simulink library "nist_library"  (R2012b)
settings: Solver=VariableStepDiscrete  StartTime=0  StopTime=1000  RelTol=1e-3
undefined symbols (not defined in the file or in its folder): sfp, xlipgetpartsetting
libraries: xbsIndex_r4 x128, xps_library x10, nist_library x5, casper_library_misc x2, casper_library_delays x1
(part 2 of 3)

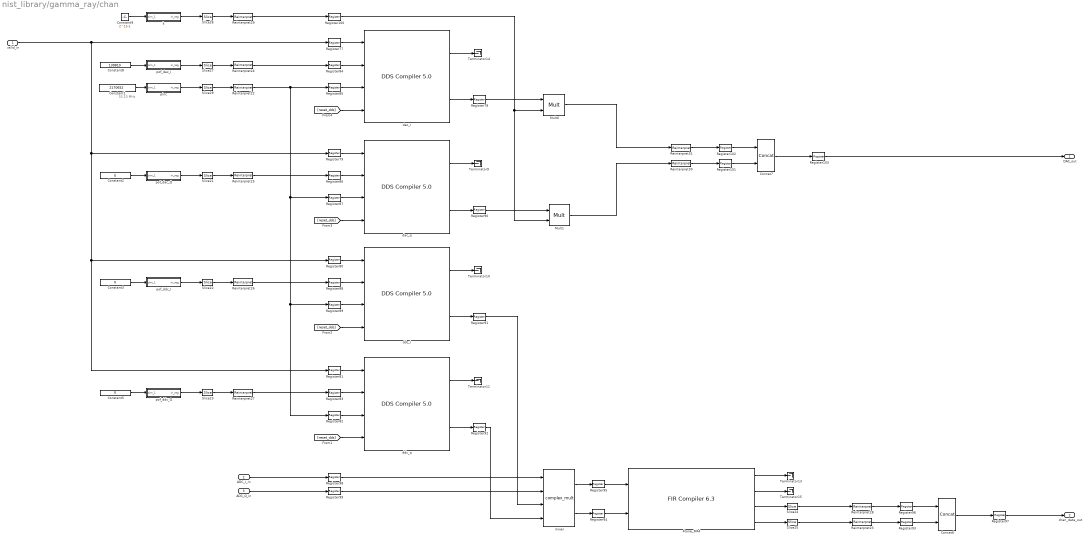
== system nist_library/gamma_ray/chan ==
  note: 33.10 MHz
  valid_in : Inport
  ADC_I_in : Inport  Port=2
  ADC_Q_in : Inport  Port=3
  4tone_FIR4 : xbsIndex_r4/FIR Compiler 6.3   coefficientvector=|  coefficient_sets=1  coefficient_reload=off  filter_type=Decimation  rate_change_type=Integer  interpolation_rate=1  decimation_rate=32  zero_pack_factor=1  channel_sequence=Basic  number_channels=1  pattern_list='P4-0,P4-1,P4-2,P4-3,P4-4'  number_paths=2  ratespecification=Maximum_Possible  sampleperiod=1  hardwareoversamplingrate=1  coefficient_sign=Signed  quantization=Maximize_Dynamic_Range  coefficient_width=14  bestprecision=on  coefficient_fractional_bits=19  coefficient_structure=Inferred  output_rounding_mode=Full_Precision  output_width=37  filter_architecture=Systolic_Multiply_Accumulate  optimization_goal=Speed  data_buffer_type=Automatic  coefficient_buffer_type=Automatic  input_buffer_type=Automatic  output_buffer_type=Automatic  preference_for_other_storage=Automatic  multi_column_support=Automatic  columnconfig='6'  inter_column_pipe_length=4  data_has_tlast=Not_Required  m_data_has_tready=off  s_data_has_fifo=off  s_data_has_tuser=Not_Required  m_data_has_tuser=Not_Required  s_config_sync_mode=On_Vector  s_config_method=Single  num_reload_slots=1  has_aclken=off  has_aresetn=off  infoeditControl=ARESETn must be asserted for a minimum of 2 cycles  trim_axipin_name=on  passband_min=0.0  passband_max=0.5  stopband_min=0.5  stopband_max=1.0  filter_selection=1  gui_behaviour=Sysgen_GUI  data_sign=Signed  data_width=16  data_fractional_bits=0  data_tuser_width=1  wrapper_available=true  ip_wrap_arbitrary_binary_point=true  ip_name=FIR Compiler  ip_version=6.3  dsptool_ready=true  ipcore_usecache=true  ipcore_useipmodelcache=true  ipcore_xco_need_fpga_part=true  port_translation_map={ 'aclken' => 'en', 'aresetn' => 'rst' }  run_core_at_system_period=true  ipcore_fpga_part=xlipgetpartsetting(gcb, {'virtex6', 'xc6vlx75t', '-3', 'ff784'})  block_type=fir_compiler_v6_3
      | [-0.004945576762396428,
      |   -0.0004342883057649687,
      |   -0.0004527757842562489,
      |   -0.00047135508794586133,
      |   -0.0004900760160352433,
      |   -0.0005088491202341634,
      |   -0.0005276998075326542,
      |   -0.000546547689892913,
      |   -0.0005654106976756595,
      |   -0.0005842536506410355,
      |   -0.0006030758678252529,
      |   -0.0006218519805181901,
      |   -0.0006405593109170567,
      |   -0.0006591567458735757,
      |   -0.0006776073739076259,
      |   -0.0006958986468812184,
      |   -0.0007140042099462066,
      |   -0.0007319006600209546,
      |   -0.0007495093972269049,
      |   -0.0007668271585960446,
      |   -0.0007837985973345622,
      |   -0.0008004847303040206,
      |   -0.000816558074371364,
      |   -0.0008326200345679305,
      |   -0.0008476890784144612,
      |   -0.0008625819845990018,
      |   -0.0008769170955610819,
      |   -0.0008905305577127275,
      |   -0.0009033656899299501,
      |   -0.0009156876002588938,
      |   -0.0009273520644178088,
      |   -0.0009382657988844351,
      |   -0.0009483110316064441,
      |   -0.0009574973347303523,
      |   -0.0009658333049719338,
      |   -0.0009733313313066214,
      |   -0.0009799587143928333,
      |   -0.0009856660600118781,
      |   -0.0009903926937808462,
      |   -0.0009940677596952641,
      |   -0.0009966598452596546,
      |   -0.000998153968519799,
      |   -0.000998593356035598,
      |   -0.0009979111825704338,
      |   -0.0009960294595758752,
      |   -0.0009926783563137058,
      |   -0.0009880436514076226,
      |   -0.000982031391898333,
      |   -0.0009746337113269129,
      |   -0.0009654980393360141,
      |   -0.0009551560082698979,
      |   -0.0009429957574212681,
      |   -0.0009294056596159474,
      |   -0.000914171602626857,
      |   -0.0008973503366857223,
      |   -0.000878942322437554,
      |   -0.000859007904965905,
      |   -0.0008375223708520817,
      |   -0.0008144740754976798,
      |   -0.0007898272475786514,
      |   -0.000763536797547961,
      |   -0.0007355014208217633,
      |   -0.0007055613466193147,
      |   -0.0006735396862409652,
      |   -0.0006392625855017414,
      |   -0.0006026653869321149,
      |   -0.0005638068586411848,
      |   -0.0005230595719924339,
      |   -0.0004809687403886442,
      |   -0.00043837704566643677,
      |   -0.00039560896213626615,
      |   -0.00035091342147599566,
      |   -0.00029119482633680816,
      |   -0.00024536833097263795,
      |   -0.0001906961065569639,
      |   -0.00013483102607781525,
      |   -0.00007690955909354745,
      |   -0.000016939572257551775,
      |   0.00004513495368569713,
      |   0.00010925887350151524,
      |   0.00017545824739311695,
      |   0.00024370647006966253,
      |   0.0003140097493414791,
      |   0.00038636169901666757,
      |   0.0004607657781277247,
      |   0.0005372061736658805,
      |   0.0006156568094935992,
      |   0.0006961175943544187,
      |   0.0007785853200736446,
      |   0.0008630788198892816,
      |   0.0009495445843636534,
      |   0.0010379964931242205,
      |   0.001128373604827996,
      |   0.0012207869406940261,
      |   0.0013147339335047488,
      |   0.0014113051117916689,
      |   0.0015088046287546986,
      |   0.0016086178618879032,
      |   0.001710374623684377,
      |   0.001813704207904973,
      |   0.001918476737258179,
      |   0.0020249986066717507,
      |   0.0021332426046828837,
      |   0.002243139281813915,
      |   0.0023545178342436524,
      |   0.002467311106773295,
      |   0.0025814917958775327,
      |   0.0026970805798065944,
      |   0.0028140764665559688,
      |   0.002932452736284891,
      |   0.003052149716212075,
      |   0.0031730589096328936,
      |   0.003295082974456467,
      |   0.0034181327776174643,
      |   0.0035422318687688874,
      |   0.0036673470602604937,
      |   0.003793474203475983,
      |   0.0039202919503391115,
      |   0.004047974298812806,
      |   0.004176310479278306,
      |   0.004305369824361406,
      |   0.004434823623226295,
      |   0.0045650237557334685,
      |   0.0046955130722802505,
      |   0.004826572927246175,
      |   0.00495798092373961,
      |   0.005089684001623189,
      |   0.005221568885099941,
      |   0.005353580377814376,
      |   0.005485579174458702,
      |   0.005617437626364228,
      |   0.005749047117597647,
      |   0.0058803760039980715,
      |   0.006011442594511834,
      |   0.006142272122013944,
      |   0.006272868641007802,
      |   0.0064031295153719504,
      |   0.006532863680215721,
      |   0.006661734821984142,
      |   0.006789525170342706,
      |   0.006916152986843038,
      |   0.0070421853694426426,
      |   0.007168266899850572,
      |   0.007294020325804492,
      |   0.0074148009918842,
      |   0.007538089119347543,
      |   0.007658471844329333,
      |   0.007777822658570999,
      |   0.007895704119665286,
      |   0.008012090275347652,
      |   0.008126861717259622,
      |   0.008239992610369232,
      |   0.008351384354342956,
      |   0.008460987880866197,
      |   0.008568730151338539,
      |   0.008674543678558294,
      |   0.008778340723400018,
      |   0.008880044308708633,
      |   0.008979602919157281,
      |   0.00907695323823665,
      |   0.00917204042884042,
      |   0.009264766789124777,
      |   0.009355105058699655,
      |   0.009442951431156595,
      |   0.009528293972594817,
      |   0.009610871314808363,
      |   0.009691496211636529,
      |   0.009767947553766466,
      |   0.009843401553078193,
      |   0.009915416541618427,
      |   0.009984126316499963,
      |   0.010050047903624215,
      |   0.010113422494991843,
      |   0.01017390543674861,
      |   0.010231296264840794,
      |   0.01028545119457461,
      |   0.010336421183108397,
      |   0.01038426038132455,
      |   0.010429014817948074,
      |   0.010470657332826963,
      |   0.01050912404868889,
      |   0.010544328818563124,
      |   0.01057618966061078,
      |   0.010604689751135063,
      |   0.010629849419136417,
      |   0.010651746091485394,
      |   0.010670350333632157,
      |   0.010685647353241094,
      |   0.010697494071983258,
      |   0.010706134504002181,
      |   0.010711226649567312,
      |   0.0107129982903304,
      |   0.010711226649567312,
      |   0.010706134504002181,
      |   0.010697494071983258,
      |   0.010685647353241094,
      |   0.010670350333632157,
      |   0.010651746091485394,
      |   0.010629849419136417,
      |   0.010604689751135063,
      |   0.01057618966061078,
      |   0.010544328818563124,
      |   0.01050912404868889,
      |   0.010470657332826963,
      |   0.010429014817948074,
      |   0.01038426038132455,
      |   0.010336421183108397,
      |   0.01028545119457461,
      |   0.010231296264840794,
      |   0.01017390543674861,
      |   0.010113422494991845,
      |   0.010050047903624215,
      |   0.009984126316499961,
      |   0.009915416541618425,
      |   0.009843401553078193,
      |   0.009767947553766466,
      |   0.009691496211636529,
      |   0.009610871314808363,
      |   0.009528293972594817,
      |   0.009442951431156595,
      |   0.009355105058699655,
      |   0.009264766789124777,
      |   0.00917204042884042,
      |   0.00907695323823665,
      |   0.008979602919157281,
      |   0.008880044308708633,
      |   0.008778340723400018,
      |   0.008674543678558294,
      |   0.008568730151338539,
      |   0.008460987880866197,
      |   0.008351384354342956,
      |   0.008239992610369232,
      |   0.008126861717259622,
      |   0.008012090275347652,
      |   0.007895704119665286,
      |   0.007777822658571,
      |   0.007658471844329333,
      |   0.007538089119347543,
      |   0.0074148009918842,
      |   0.007294020325804492,
      |   0.007168266899850572,
      |   0.0070421853694426426,
      |   0.006916152986843038,
      |   0.006789525170342706,
      |   0.006661734821984142,
      |   0.006532863680215721,
      |   0.0064031295153719504,
      |   0.006272868641007802,
      |   0.006142272122013944,
      |   0.006011442594511834,
      |   0.0058803760039980715,
      |   0.005749047117597647,
      |   0.005617437626364228,
      |   0.005485579174458702,
      |   0.005353580377814376,
      |   0.005221568885099941,
      |   0.005089684001623189,
      |   0.00495798092373961,
      |   0.004826572927246175,
      |   0.0046955130722802505,
      |   0.0045650237557334685,
      |   0.004434823623226295,
      |   0.004305369824361406,
      |   0.004176310479278306,
      |   0.004047974298812806,
      |   0.0039202919503391115,
      |   0.003793474203475983,
      |   0.0036673470602604937,
      |   0.0035422318687688874,
      |   0.0034181327776174647,
      |   0.003295082974456466,
      |   0.0031730589096328936,
      |   0.003052149716212075,
      |   0.002932452736284891,
      |   0.0028140764665559688,
      |   0.0026970805798065944,
      |   0.0025814917958775327,
      |   0.002467311106773295,
      |   0.0023545178342436524,
      |   0.002243139281813915,
      |   0.0021332426046828837,
      |   0.0020249986066717507,
      |   0.0019184767372581789,
      |   0.0018137042079049725,
      |   0.001710374623684377,
      |   0.0016086178618879032,
      |   0.0015088046287546986,
      |   0.0014113051117916689,
      |   0.0013147339335047488,
      |   0.0012207869406940261,
      |   0.001128373604827996,
      |   0.0010379964931242205,
      |   0.0009495445843636534,
      |   0.0008630788198892816,
      |   0.0007785853200736446,
      |   0.0006961175943544187,
      |   0.0006156568094935992,
      |   0.0005372061736658805,
      |   0.0004607657781277247,
      |   0.00038636169901666757,
      |   0.0003140097493414791,
      |   0.00024370647006966253,
      |   0.000175458247393117,
      |   0.00010925887350151526,
      |   0.000045134953685697144,
      |   -0.000016939572257551775,
      |   -0.00007690955909354741,
      |   -0.00013483102607781503,
      |   -0.0001906961065569639,
      |   -0.00024536833097263795,
      |   -0.00029119482633680816,
      |   -0.0003509134214759956,
      |   -0.00039560896213626615,
      |   -0.00043837704566643677,
      |   -0.0004809687403886442,
      |   -0.0005230595719924339,
      |   -0.0005638068586411848,
      |   -0.0006026653869321149,
      |   -0.0006392625855017414,
      |   -0.0006735396862409652,
      |   -0.0007055613466193147,
      |   -0.0007355014208217633,
      |   -0.000763536797547961,
      |   -0.000789827247578651,
      |   -0.0008144740754976798,
      |   -0.0008375223708520817,
      |   -0.000859007904965905,
      |   -0.000878942322437554,
      |   -0.0008973503366857223,
      |   -0.000914171602626857,
      |   -0.0009294056596159474,
      |   -0.0009429957574212681,
      |   -0.0009551560082698979,
      |   -0.0009654980393360141,
      |   -0.0009746337113269129,
      |   -0.000982031391898333,
      |   -0.0009880436514076226,
      |   -0.0009926783563137065,
      |   -0.0009960294595758755,
      |   -0.0009979111825704338,
      |   -0.000998593356035598,
      |   -0.0009981539685197994,
      |   -0.0009966598452596546,
      |   -0.0009940677596952641,
      |   -0.0009903926937808462,
      |   -0.000985666060011878,
      |   -0.0009799587143928333,
      |   -0.0009733313313066214,
      |   -0.0009658333049719338,
      |   -0.0009574973347303529,
      |   -0.0009483110316064446,
      |   -0.0009382657988844346,
      |   -0.0009273520644178088,
      |   -0.0009156876002588938,
      |   -0.0009033656899299501,
      |   -0.0008905305577127275,
      |   -0.0008769170955610819,
      |   -0.0008625819845990029,
      |   -0.0008476890784144612,
      |   -0.0008326200345679302,
      |   -0.000816558074371364,
      |   -0.0008004847303040206,
      |   -0.0007837985973345619,
      |   -0.0007668271585960446,
      |   -0.0007495093972269048,
      |   -0.0007319006600209546,
      |   -0.000714004209946207,
      |   -0.0006958986468812184,
      |   -0.0006776073739076259,
      |   -0.0006591567458735757,
      |   -0.0006405593109170567,
      |   -0.0006218519805181902,
      |   -0.0006030758678252529,
      |   -0.0005842536506410353,
      |   -0.0005654106976756595,
      |   -0.000546547689892913,
      |   -0.0005276998075326542,
      |   -0.0005088491202341634,
      |   -0.0004900760160352433,
      |   -0.00047135508794586133,
      |   -0.0004527757842562489,
      |   -0.0004342883057649687,
      |   -0.004945576762396428]
      settings: infoedit=Maximum Possible : Maximizes oversampling rate. Abstracted input handshake (no s_data_tvalid) and automatic rate propagation.<br>Hardware Oversampling Rate : Specifies oversampling rate relative to the input sample period. Abstracted input handshake (no s_data_tvalid) and automatic rate propagation.<br>Sample Period : Specifies absolute oversampling rate. No input handshake abstraction (exposes s_data_tvalid) and no rate propagation.
  Concat6 : xbsIndex_r4/Concat  num_inputs=2  dbl_ovrd=off  block_type=concat
  Concat7 : xbsIndex_r4/Concat  num_inputs=2  dbl_ovrd=off  block_type=concat
  Constant1 : Constant  Value=2170652
  Constant2 : Constant  Value=0
  Constant3 : Constant  Value=0
  Constant5 : Constant  Value=0
  Constant8 : Constant  Value=139810
  Constant9 : Constant  Value=2^15-1
  Mult0 : xbsIndex_r4/Mult  precision=User Defined  arith_type="Signed  (2's comp)"  n_bits=16  bin_pt=15  quantization=Truncate  overflow=Wrap  en=off  latency=4  dbl_ovrd=off  use_behavioral_HDL=off  opt=Speed  use_embedded=on  optimum_pipeline=off  pipeline=on  use_rpm=on  placement_style=Triangular  block_type=mult
  Mult1 : xbsIndex_r4/Mult  precision=User Defined  arith_type="Signed  (2's comp)"  n_bits=16  bin_pt=15  quantization=Truncate  overflow=Wrap  en=off  latency=4  dbl_ovrd=off  use_behavioral_HDL=off  opt=Speed  use_embedded=on  optimum_pipeline=off  pipeline=on  use_rpm=on  placement_style=Triangular  block_type=mult
  Register{77..103} (27 alike) : xbsIndex_r4/Register  init=0  rst=off  en=off  dbl_ovrd=off  block_type=register
  Reinterpret{22,24..27} (5 alike) : xbsIndex_r4/Reinterpret  force_arith_type=on  arith_type="Signed  (2's comp)"  force_bin_pt=on  bin_pt=24  block_type=reinterpret
      settings: block_version=10.1.3
  Reinterpret{23,28,30..31} (4 alike) : xbsIndex_r4/Reinterpret  force_arith_type=on  arith_type=Unsigned  force_bin_pt=on  bin_pt=0  block_type=reinterpret
      settings: block_version=10.1.3
  Reinterpret29 : xbsIndex_r4/Reinterpret  force_arith_type=on  arith_type="Signed  (2's comp)"  force_bin_pt=on  bin_pt=15  block_type=reinterpret
      settings: block_version=10.1.3
  Slice{21..23,27,29} (5 alike) : xbsIndex_r4/Slice  nbits=24  boolean_output=off  mode=Lower Bit Location + Width  bit1=0  base1=MSB of Input  bit0=0  base0=LSB of Input  dbl_ovrd=off  block_type=slice
      settings: block_version=10.1.3
  Slice24 : xbsIndex_r4/Slice  nbits=32  boolean_output=off  mode=Two Bit Locations  bit1=2  base1=Binary Point of Input  bit0=-16  base0=Binary Point of Input  dbl_ovrd=off  block_type=slice
      settings: block_version=10.1.3
  Slice25 : xbsIndex_r4/Slice  nbits=32  boolean_output=off  mode=Two Bit Locations  bit1=2  base1=Binary Point of Input  bit0=-16  base0=Binary Point of Input  dbl_ovrd=off  block_type=slice
      settings: block_version=10.1.3
  Slice26 : xbsIndex_r4/Slice  nbits=16  boolean_output=off  mode=Lower Bit Location + Width  bit1=0  base1=MSB of Input  bit0=0  base0=LSB of Input  dbl_ovrd=off  block_type=slice
      settings: block_version=10.1.3
  Terminator{9..11,13..15} (6 alike) : Terminator
  dac_I : xbsIndex_r4/DDS Compiler 5.0   partspresent=Phase_Generator_and_SIN_COS_LUT  dds_clock_rate=256  channels=1  parameter_entry=Hardware_Parameters  spurious_free_dynamic_range=36  frequency_resolution=0.4  noise_shaping=None  phase_width=24  output_width=16  output_selection=Cosine  negative_sine=off  negative_cosine=off  amplitude_mode=Full_Range  memory_type=Auto  optimization_goal=Speed  dsp48_use=Maximal  latency_configuration=Auto  latency=5  has_phase_out=off  has_aclken=off  has_aresetn=on  explicit_period=off  period=1  data_has_tlast=Not_Required  has_tready=off  s_phase_has_tuser=Not_Required  m_data_has_tuser=Not_Required  m_phase_has_tuser=Not_Required  s_phase_tuser_width=1  s_config_sync_mode=On_Vector  phase_increment=Programmable  output_frequency1=0  output_frequency2=0  output_frequency3=0  output_frequency4=0  output_frequency5=0  output_frequency6=0  output_frequency7=0  output_frequency8=0  output_frequency9=0  output_frequency10=0  output_frequency11=0  output_frequency12=0  output_frequency13=0  output_frequency14=0  output_frequency15=0  output_frequency16=0  pinc1='1101000110110'  pinc2='0'  pinc3='0'  pinc4='0'  pinc5='0'  pinc6='0'  pinc7='0'  pinc8='0'  pinc9='0'  pinc10='0'  pinc11='0'  pinc12='0'  pinc13='0'  pinc14='0'  pinc15='0'  pinc16='0'  phase_offset=Programmable  phase_offset_angles1=0  phase_offset_angles2=0  phase_offset_angles3=0  phase_offset_angles4=0  phase_offset_angles5=0  phase_offset_angles6=0  phase_offset_angles7=0  phase_offset_angles8=0  phase_offset_angles9=0  phase_offset_angles10=0  phase_offset_angles11=0  phase_offset_angles12=0  phase_offset_angles13=0  phase_offset_angles14=0  phase_offset_angles15=0  phase_offset_angles16=0  poff1='0'  poff2='0'  poff3='0'  poff4='0'  poff5='0'  poff6='0'  poff7='0'  poff8='0'  poff9='0'  poff10='0'  poff11='0'  poff12='0'  poff13='0'  poff14='0'  poff15='0'  poff16='0'  trim_axipin_name=on  por_mode=false  gui_behaviour=Sysgen  ip_name=DDS Compiler  ip_version=5.0  dsptool_ready=true  wrapper_available=true  port_translation_map={ 'aclken' => 'en', 'aresetn' => 'rst' }  ipcore_xco_need_fpga_part=true  ipcore_fpga_part=xlipgetpartsetting(gcb, {'virtex6', 'xc6vlx75t', '-3', 'ff784'})  ipcore_usecache=true  ipcore_useipmodelcache=true  ipcore_verbose=false  block_type=dds_compiler_v5_0
  dac_q : xbsIndex_r4/DDS Compiler 5.0   partspresent=Phase_Generator_and_SIN_COS_LUT  dds_clock_rate=256  channels=1  parameter_entry=Hardware_Parameters  spurious_free_dynamic_range=36  frequency_resolution=0.4  noise_shaping=None  phase_width=24  output_width=16  output_selection=Cosine  negative_sine=off  negative_cosine=off  amplitude_mode=Full_Range  memory_type=Auto  optimization_goal=Speed  dsp48_use=Maximal  latency_configuration=Auto  latency=5  has_phase_out=off  has_aclken=off  has_aresetn=on  explicit_period=off  period=1  data_has_tlast=Not_Required  has_tready=off  s_phase_has_tuser=Not_Required  m_data_has_tuser=Not_Required  m_phase_has_tuser=Not_Required  s_phase_tuser_width=1  s_config_sync_mode=On_Vector  phase_increment=Programmable  output_frequency1=0  output_frequency2=0  output_frequency3=0  output_frequency4=0  output_frequency5=0  output_frequency6=0  output_frequency7=0  output_frequency8=0  output_frequency9=0  output_frequency10=0  output_frequency11=0  output_frequency12=0  output_frequency13=0  output_frequency14=0  output_frequency15=0  output_frequency16=0  pinc1='1101000110110'  pinc2='0'  pinc3='0'  pinc4='0'  pinc5='0'  pinc6='0'  pinc7='0'  pinc8='0'  pinc9='0'  pinc10='0'  pinc11='0'  pinc12='0'  pinc13='0'  pinc14='0'  pinc15='0'  pinc16='0'  phase_offset=Programmable  phase_offset_angles1=0  phase_offset_angles2=0  phase_offset_angles3=0  phase_offset_angles4=0  phase_offset_angles5=0  phase_offset_angles6=0  phase_offset_angles7=0  phase_offset_angles8=0  phase_offset_angles9=0  phase_offset_angles10=0  phase_offset_angles11=0  phase_offset_angles12=0  phase_offset_angles13=0  phase_offset_angles14=0  phase_offset_angles15=0  phase_offset_angles16=0  poff1='0'  poff2='0'  poff3='0'  poff4='0'  poff5='0'  poff6='0'  poff7='0'  poff8='0'  poff9='0'  poff10='0'  poff11='0'  poff12='0'  poff13='0'  poff14='0'  poff15='0'  poff16='0'  trim_axipin_name=on  por_mode=false  gui_behaviour=Sysgen  ip_name=DDS Compiler  ip_version=5.0  dsptool_ready=true  wrapper_available=true  port_translation_map={ 'aclken' => 'en', 'aresetn' => 'rst' }  ipcore_xco_need_fpga_part=true  ipcore_fpga_part=xlipgetpartsetting(gcb, {'virtex6', 'xc6vlx75t', '-3', 'ff784'})  ipcore_usecache=true  ipcore_useipmodelcache=true  ipcore_verbose=false  block_type=dds_compiler_v5_0
  ddc_I : xbsIndex_r4/DDS Compiler 5.0   partspresent=Phase_Generator_and_SIN_COS_LUT  dds_clock_rate=256  channels=1  parameter_entry=Hardware_Parameters  spurious_free_dynamic_range=36  frequency_resolution=0.4  noise_shaping=None  phase_width=24  output_width=12  output_selection=Cosine  negative_sine=off  negative_cosine=off  amplitude_mode=Full_Range  memory_type=Auto  optimization_goal=Speed  dsp48_use=Maximal  latency_configuration=Auto  latency=9  has_phase_out=off  has_aclken=off  has_aresetn=on  explicit_period=off  period=1  data_has_tlast=Not_Required  has_tready=off  s_phase_has_tuser=Not_Required  m_data_has_tuser=Not_Required  m_phase_has_tuser=Not_Required  s_phase_tuser_width=1  s_config_sync_mode=On_Vector  phase_increment=Programmable  output_frequency1=0  output_frequency2=0  output_frequency3=0  output_frequency4=0  output_frequency5=0  output_frequency6=0  output_frequency7=0  output_frequency8=0  output_frequency9=0  output_frequency10=0  output_frequency11=0  output_frequency12=0  output_frequency13=0  output_frequency14=0  output_frequency15=0  output_frequency16=0  pinc1='1101000110110'  pinc2='0'  pinc3='0'  pinc4='0'  pinc5='0'  pinc6='0'  pinc7='0'  pinc8='0'  pinc9='0'  pinc10='0'  pinc11='0'  pinc12='0'  pinc13='0'  pinc14='0'  pinc15='0'  pinc16='0'  phase_offset=Programmable  phase_offset_angles1=0  phase_offset_angles2=0  phase_offset_angles3=0  phase_offset_angles4=0  phase_offset_angles5=0  phase_offset_angles6=0  phase_offset_angles7=0  phase_offset_angles8=0  phase_offset_angles9=0  phase_offset_angles10=0  phase_offset_angles11=0  phase_offset_angles12=0  phase_offset_angles13=0  phase_offset_angles14=0  phase_offset_angles15=0  phase_offset_angles16=0  poff1='0'  poff2='0'  poff3='0'  poff4='0'  poff5='0'  poff6='0'  poff7='0'  poff8='0'  poff9='0'  poff10='0'  poff11='0'  poff12='0'  poff13='0'  poff14='0'  poff15='0'  poff16='0'  trim_axipin_name=on  por_mode=false  gui_behaviour=Sysgen  ip_name=DDS Compiler  ip_version=5.0  dsptool_ready=true  wrapper_available=true  port_translation_map={ 'aclken' => 'en', 'aresetn' => 'rst' }  ipcore_xco_need_fpga_part=true  ipcore_fpga_part=xlipgetpartsetting(gcb, {'virtex6', 'xc6vlx75t', '-3', 'ff784'})  ipcore_usecache=true  ipcore_useipmodelcache=true  ipcore_verbose=false  block_type=dds_compiler_v5_0
  ddc_q : xbsIndex_r4/DDS Compiler 5.0   partspresent=Phase_Generator_and_SIN_COS_LUT  dds_clock_rate=256  channels=1  parameter_entry=Hardware_Parameters  spurious_free_dynamic_range=36  frequency_resolution=0.4  noise_shaping=None  phase_width=24  output_width=12  output_selection=Cosine  negative_sine=off  negative_cosine=off  amplitude_mode=Full_Range  memory_type=Auto  optimization_goal=Speed  dsp48_use=Maximal  latency_configuration=Auto  latency=9  has_phase_out=off  has_aclken=off  has_aresetn=on  explicit_period=off  period=1  data_has_tlast=Not_Required  has_tready=off  s_phase_has_tuser=Not_Required  m_data_has_tuser=Not_Required  m_phase_has_tuser=Not_Required  s_phase_tuser_width=1  s_config_sync_mode=On_Vector  phase_increment=Programmable  output_frequency1=0  output_frequency2=0  output_frequency3=0  output_frequency4=0  output_frequency5=0  output_frequency6=0  output_frequency7=0  output_frequency8=0  output_frequency9=0  output_frequency10=0  output_frequency11=0  output_frequency12=0  output_frequency13=0  output_frequency14=0  output_frequency15=0  output_frequency16=0  pinc1='1101000110110'  pinc2='0'  pinc3='0'  pinc4='0'  pinc5='0'  pinc6='0'  pinc7='0'  pinc8='0'  pinc9='0'  pinc10='0'  pinc11='0'  pinc12='0'  pinc13='0'  pinc14='0'  pinc15='0'  pinc16='0'  phase_offset=Programmable  phase_offset_angles1=0  phase_offset_angles2=0  phase_offset_angles3=0  phase_offset_angles4=0  phase_offset_angles5=0  phase_offset_angles6=0  phase_offset_angles7=0  phase_offset_angles8=0  phase_offset_angles9=0  phase_offset_angles10=0  phase_offset_angles11=0  phase_offset_angles12=0  phase_offset_angles13=0  phase_offset_angles14=0  phase_offset_angles15=0  phase_offset_angles16=0  poff1='0'  poff2='0'  poff3='0'  poff4='0'  poff5='0'  poff6='0'  poff7='0'  poff8='0'  poff9='0'  poff10='0'  poff11='0'  poff12='0'  poff13='0'  poff14='0'  poff15='0'  poff16='0'  trim_axipin_name=on  por_mode=false  gui_behaviour=Sysgen  ip_name=DDS Compiler  ip_version=5.0  dsptool_ready=true  wrapper_available=true  port_translation_map={ 'aclken' => 'en', 'aresetn' => 'rst' }  ipcore_xco_need_fpga_part=true  ipcore_fpga_part=xlipgetpartsetting(gcb, {'virtex6', 'xc6vlx75t', '-3', 'ff784'})  ipcore_usecache=true  ipcore_useipmodelcache=true  ipcore_verbose=false  block_type=dds_compiler_v5_0
  k : Subsystem  Tag=xps:sw_reg  AncestorBlock=xps_library/software register  mask(swreg){mode=one value, io_dir=From Processor, io_delay=0, sample_period=1, names=reg, bitwidths=32, arith_types=0, bin_pts=0, sim_port=on, show_format=off}
      mask prompts: io_dir "I/O direction"; io_delay "I/O delay"; sample_period "Sample period"; names "Name:"; bitwidths "Bitwidth:"; arith_types "Type (ufix=0, fix=1, bool=2):"; bin_pts "Binary pt:"; sim_port "Provide sim input/output?"; show_format "Print format string?"
      mask init:
      | swreg_init(gcb)
      settings: AttributesFormatString=1input
      mask TypeOptions mode: one value | fields of equal size | fields of arbitrary size
      mask Callback mode: swreg_cb(gcb);
      mask TypeOptions io_dir: To Processor | From Processor
      mask Callback io_dir:
      | mask_enables = get_param(gcb, 'MaskEnables');
      | mask_names = get_param(gcb, 'MaskNames');
      | if strcmp(get_param(gcb, 'io_dir'), 'To Processor'),
      |     mask_enables{ismember(mask_names, 'sample_period')} = 'off';
      | else
      |     mask_enables{ismember(mask_names, 'sample_period')} = 'on';
      | end
      | set_param(gcb, 'MaskEnables', mask_enables);
      mask Callback bitwidths:
      | swreg_maskcheck(gcb);
      | % blk = gcb;
      | % mode = get_param(blk, 'mode');
      | % current_widths = eval(get_param(blk, 'bitwidths'));
      | % if (strcmp(mode, 'one value') || strcmp(mode, 'fields of equal size')) && (length(current_widths) > 1),
      | %     error('Only one width may be specified for this mode.');
      | % elseif strcmp(mode, 'fields of arbitrary size')
      | %     current_names = textscan(strtrim(strrep(strrep(get_param(blk, 'names'), ']', ''), '[', '')), '%s');
      | %     current_names = current_names{1};
      | %     numios = length(current_names);
      | %     if length(current_widths) ~= numios,
      | %         error('%d field names specified, but %d widths?', numios, length(current_widths));
      | %     end
      | % end
      | % total_width = 0;
      | % for ctr = 1 : length(current_widths),
      | %     total_width = total_width + current_widths(ctr);
      | % end
      | % if total_width > 32,
      | %     error('Total width must be 32 or less, set to %d.', total_width);
      | % end
      mask Callback arith_types:
      | [numios, ~, ~, ~, current_types] = swreg_maskcheck(gcb);
      | % blk = gcb;
      | % mode = get_param(blk, 'mode');
      | % current_types = eval(get_param(blk, 'arith_types'));
      | % numios = length(current_types);
      | % if (strcmp(mode, 'one value') || strcmp(mode, 'fields of equal size')) && (length(current_types) > 1),
      | %     error('Only one type may be specified for this mode.');
      | % elseif strcmp(mode, 'fields of arbitrary size')
      | %     current_names = textscan(strtrim(strrep(strrep(get_param(blk, 'names'), ']', ''), '[', '')), '%s');
      | %     current_names = current_names{1};
      | %     numios = length(current_names);
      | %     if length(current_types) ~= numios,
      | %         error('%d field names specified, but %d types?', numios, length(current_types));
      | %     end
      | % end
      | problem = 0;
      | for ctr = 1 : numios,
      |     t = current_types(ctr);
      |     if (t < 0) || (t > 2),
      |         problem = t;
      |         ctr = numios + 1;
      |     end
      | end
      | if problem ~= 0,
      |     error('Type cannot be %i, must be 0, 1 or 2.', problem);
      | end
      mask Callback bin_pts:
      | swreg_maskcheck(gcb);
      | % blk = gcb;
      | % mode = get_param(blk, 'mode');
      | % current_bins = eval(get_param(blk, 'bin_pts'));
      | % if (strcmp(mode, 'one value') || strcmp(mode, 'fields of equal size')) && (length(current_bins) > 1),
      | %     error('Only one binary pt may be specified for this mode.');
      | % elseif strcmp(mode, 'fields of arbitrary size')
      | %     current_names = textscan(strtrim(strrep(strrep(get_param(blk, 'names'), ']', ''), '[', '')), '%s');
      | %     current_names = current_names{1};
      | %     numios = length(current_names);
      | %     if length(current_bins) ~= numios,
      | %         error('%d field names specified, but %d binary pts?', numios, length(current_bins));
      | %     end
      | % end
  mixer : nist_library/complex_mult
  pinc : Subsystem  Tag=xps:sw_reg  AncestorBlock=xps_library/software register  mask(swreg){mode=one value, io_dir=From Processor, io_delay=0, sample_period=1, names=reg, bitwidths=32, arith_types=0, bin_pts=0, sim_port=on, show_format=off}
      mask prompts: io_dir "I/O direction"; io_delay "I/O delay"; sample_period "Sample period"; names "Name:"; bitwidths "Bitwidth:"; arith_types "Type (ufix=0, fix=1, bool=2):"; bin_pts "Binary pt:"; sim_port "Provide sim input/output?"; show_format "Print format string?"
      mask init:
      | swreg_init(gcb)
      settings: AttributesFormatString=1input
      mask TypeOptions mode: one value | fields of equal size | fields of arbitrary size
      mask Callback mode: swreg_cb(gcb);
      mask TypeOptions io_dir: To Processor | From Processor
      mask Callback io_dir:
      | mask_enables = get_param(gcb, 'MaskEnables');
      | mask_names = get_param(gcb, 'MaskNames');
      | if strcmp(get_param(gcb, 'io_dir'), 'To Processor'),
      |     mask_enables{ismember(mask_names, 'sample_period')} = 'off';
      | else
      |     mask_enables{ismember(mask_names, 'sample_period')} = 'on';
      | end
      | set_param(gcb, 'MaskEnables', mask_enables);
      mask Callback bitwidths:
      | swreg_maskcheck(gcb);
      | % blk = gcb;
      | % mode = get_param(blk, 'mode');
      | % current_widths = eval(get_param(blk, 'bitwidths'));
      | % if (strcmp(mode, 'one value') || strcmp(mode, 'fields of equal size')) && (length(current_widths) > 1),
      | %     error('Only one width may be specified for this mode.');
      | % elseif strcmp(mode, 'fields of arbitrary size')
      | %     current_names = textscan(strtrim(strrep(strrep(get_param(blk, 'names'), ']', ''), '[', '')), '%s');
      | %     current_names = current_names{1};
      | %     numios = length(current_names);
      | %     if length(current_widths) ~= numios,
      | %         error('%d field names specified, but %d widths?', numios, length(current_widths));
      | %     end
      | % end
      | % total_width = 0;
      | % for ctr = 1 : length(current_widths),
      | %     total_width = total_width + current_widths(ctr);
      | % end
      | % if total_width > 32,
      | %     error('Total width must be 32 or less, set to %d.', total_width);
      | % end
      mask Callback arith_types:
      | [numios, ~, ~, ~, current_types] = swreg_maskcheck(gcb);
      | % blk = gcb;
      | % mode = get_param(blk, 'mode');
      | % current_types = eval(get_param(blk, 'arith_types'));
      | % numios = length(current_types);
      | % if (strcmp(mode, 'one value') || strcmp(mode, 'fields of equal size')) && (length(current_types) > 1),
      | %     error('Only one type may be specified for this mode.');
      | % elseif strcmp(mode, 'fields of arbitrary size')
      | %     current_names = textscan(strtrim(strrep(strrep(get_param(blk, 'names'), ']', ''), '[', '')), '%s');
      | %     current_names = current_names{1};
      | %     numios = length(current_names);
      | %     if length(current_types) ~= numios,
      | %         error('%d field names specified, but %d types?', numios, length(current_types));
      | %     end
      | % end
      | problem = 0;
      | for ctr = 1 : numios,
      |     t = current_types(ctr);
      |     if (t < 0) || (t > 2),
      |         problem = t;
      |         ctr = numios + 1;
      |     end
      | end
      | if problem ~= 0,
      |     error('Type cannot be %i, must be 0, 1 or 2.', problem);
      | end
      mask Callback bin_pts:
      | swreg_maskcheck(gcb);
      | % blk = gcb;
      | % mode = get_param(blk, 'mode');
      | % current_bins = eval(get_param(blk, 'bin_pts'));
      | % if (strcmp(mode, 'one value') || strcmp(mode, 'fields of equal size')) && (length(current_bins) > 1),
      | %     error('Only one binary pt may be specified for this mode.');
      | % elseif strcmp(mode, 'fields of arbitrary size')
      | %     current_names = textscan(strtrim(strrep(strrep(get_param(blk, 'names'), ']', ''), '[', '')), '%s');
      | %     current_names = current_names{1};
      | %     numios = length(current_names);
      | %     if length(current_bins) ~= numios,
      | %         error('%d field names specified, but %d binary pts?', numios, length(current_bins));
      | %     end
      | % end
  pof_dac_I : Subsystem  Tag=xps:sw_reg  AncestorBlock=xps_library/software register  mask(swreg){mode=one value, io_dir=From Processor, io_delay=0, sample_period=1, names=reg, bitwidths=32, arith_types=0, bin_pts=0, sim_port=on, show_format=off}
      mask prompts: io_dir "I/O direction"; io_delay "I/O delay"; sample_period "Sample period"; names "Name:"; bitwidths "Bitwidth:"; arith_types "Type (ufix=0, fix=1, bool=2):"; bin_pts "Binary pt:"; sim_port "Provide sim input/output?"; show_format "Print format string?"
      mask init:
      | swreg_init(gcb)
      settings: AttributesFormatString=1input
      mask TypeOptions mode: one value | fields of equal size | fields of arbitrary size
      mask Callback mode: swreg_cb(gcb);
      mask TypeOptions io_dir: To Processor | From Processor
      mask Callback io_dir:
      | mask_enables = get_param(gcb, 'MaskEnables');
      | mask_names = get_param(gcb, 'MaskNames');
      | if strcmp(get_param(gcb, 'io_dir'), 'To Processor'),
      |     mask_enables{ismember(mask_names, 'sample_period')} = 'off';
      | else
      |     mask_enables{ismember(mask_names, 'sample_period')} = 'on';
      | end
      | set_param(gcb, 'MaskEnables', mask_enables);
      mask Callback bitwidths:
      | swreg_maskcheck(gcb);
      | % blk = gcb;
      | % mode = get_param(blk, 'mode');
      | % current_widths = eval(get_param(blk, 'bitwidths'));
      | % if (strcmp(mode, 'one value') || strcmp(mode, 'fields of equal size')) && (length(current_widths) > 1),
      | %     error('Only one width may be specified for this mode.');
      | % elseif strcmp(mode, 'fields of arbitrary size')
      | %     current_names = textscan(strtrim(strrep(strrep(get_param(blk, 'names'), ']', ''), '[', '')), '%s');
      | %     current_names = current_names{1};
      | %     numios = length(current_names);
      | %     if length(current_widths) ~= numios,
      | %         error('%d field names specified, but %d widths?', numios, length(current_widths));
      | %     end
      | % end
      | % total_width = 0;
      | % for ctr = 1 : length(current_widths),
      | %     total_width = total_width + current_widths(ctr);
      | % end
      | % if total_width > 32,
      | %     error('Total width must be 32 or less, set to %d.', total_width);
      | % end
      mask Callback arith_types:
      | [numios, ~, ~, ~, current_types] = swreg_maskcheck(gcb);
      | % blk = gcb;
      | % mode = get_param(blk, 'mode');
      | % current_types = eval(get_param(blk, 'arith_types'));
      | % numios = length(current_types);
      | % if (strcmp(mode, 'one value') || strcmp(mode, 'fields of equal size')) && (length(current_types) > 1),
      | %     error('Only one type may be specified for this mode.');
      | % elseif strcmp(mode, 'fields of arbitrary size')
      | %     current_names = textscan(strtrim(strrep(strrep(get_param(blk, 'names'), ']', ''), '[', '')), '%s');
      | %     current_names = current_names{1};
      | %     numios = length(current_names);
      | %     if length(current_types) ~= numios,
      | %         error('%d field names specified, but %d types?', numios, length(current_types));
      | %     end
      | % end
      | problem = 0;
      | for ctr = 1 : numios,
      |     t = current_types(ctr);
      |     if (t < 0) || (t > 2),
      |         problem = t;
      |         ctr = numios + 1;
      |     end
      | end
      | if problem ~= 0,
      |     error('Type cannot be %i, must be 0, 1 or 2.', problem);
      | end
      mask Callback bin_pts:
      | swreg_maskcheck(gcb);
      | % blk = gcb;
      | % mode = get_param(blk, 'mode');
      | % current_bins = eval(get_param(blk, 'bin_pts'));
      | % if (strcmp(mode, 'one value') || strcmp(mode, 'fields of equal size')) && (length(current_bins) > 1),
      | %     error('Only one binary pt may be specified for this mode.');
      | % elseif strcmp(mode, 'fields of arbitrary size')
      | %     current_names = textscan(strtrim(strrep(strrep(get_param(blk, 'names'), ']', ''), '[', '')), '%s');
      | %     current_names = current_names{1};
      | %     numios = length(current_names);
      | %     if length(current_bins) ~= numios,
      | %         error('%d field names specified, but %d binary pts?', numios, length(current_bins));
      | %     end
      | % end
  pof_dac_Q : Subsystem  Tag=xps:sw_reg  AncestorBlock=xps_library/software register  mask(swreg){mode=one value, io_dir=From Processor, io_delay=0, sample_period=1, names=reg, bitwidths=32, arith_types=0, bin_pts=0, sim_port=on, show_format=off}
      mask prompts: io_dir "I/O direction"; io_delay "I/O delay"; sample_period "Sample period"; names "Name:"; bitwidths "Bitwidth:"; arith_types "Type (ufix=0, fix=1, bool=2):"; bin_pts "Binary pt:"; sim_port "Provide sim input/output?"; show_format "Print format string?"
      mask init:
      | swreg_init(gcb)
      settings: AttributesFormatString=1input
      mask TypeOptions mode: one value | fields of equal size | fields of arbitrary size
      mask Callback mode: swreg_cb(gcb);
      mask TypeOptions io_dir: To Processor | From Processor
      mask Callback io_dir:
      | mask_enables = get_param(gcb, 'MaskEnables');
      | mask_names = get_param(gcb, 'MaskNames');
      | if strcmp(get_param(gcb, 'io_dir'), 'To Processor'),
      |     mask_enables{ismember(mask_names, 'sample_period')} = 'off';
      | else
      |     mask_enables{ismember(mask_names, 'sample_period')} = 'on';
      | end
      | set_param(gcb, 'MaskEnables', mask_enables);
      mask Callback bitwidths:
      | swreg_maskcheck(gcb);
      | % blk = gcb;
      | % mode = get_param(blk, 'mode');
      | % current_widths = eval(get_param(blk, 'bitwidths'));
      | % if (strcmp(mode, 'one value') || strcmp(mode, 'fields of equal size')) && (length(current_widths) > 1),
      | %     error('Only one width may be specified for this mode.');
      | % elseif strcmp(mode, 'fields of arbitrary size')
      | %     current_names = textscan(strtrim(strrep(strrep(get_param(blk, 'names'), ']', ''), '[', '')), '%s');
      | %     current_names = current_names{1};
      | %     numios = length(current_names);
      | %     if length(current_widths) ~= numios,
      | %         error('%d field names specified, but %d widths?', numios, length(current_widths));
      | %     end
      | % end
      | % total_width = 0;
      | % for ctr = 1 : length(current_widths),
      | %     total_width = total_width + current_widths(ctr);
      | % end
      | % if total_width > 32,
      | %     error('Total width must be 32 or less, set to %d.', total_width);
      | % end
      mask Callback arith_types:
      | [numios, ~, ~, ~, current_types] = swreg_maskcheck(gcb);
      | % blk = gcb;
      | % mode = get_param(blk, 'mode');
      | % current_types = eval(get_param(blk, 'arith_types'));
      | % numios = length(current_types);
      | % if (strcmp(mode, 'one value') || strcmp(mode, 'fields of equal size')) && (length(current_types) > 1),
      | %     error('Only one type may be specified for this mode.');
      | % elseif strcmp(mode, 'fields of arbitrary size')
      | %     current_names = textscan(strtrim(strrep(strrep(get_param(blk, 'names'), ']', ''), '[', '')), '%s');
      | %     current_names = current_names{1};
      | %     numios = length(current_names);
      | %     if length(current_types) ~= numios,
      | %         error('%d field names specified, but %d types?', numios, length(current_types));
      | %     end
      | % end
      | problem = 0;
      | for ctr = 1 : numios,
      |     t = current_types(ctr);
      |     if (t < 0) || (t > 2),
      |         problem = t;
      |         ctr = numios + 1;
      |     end
      | end
      | if problem ~= 0,
      |     error('Type cannot be %i, must be 0, 1 or 2.', problem);
      | end
      mask Callback bin_pts:
      | swreg_maskcheck(gcb);
      | % blk = gcb;
      | % mode = get_param(blk, 'mode');
      | % current_bins = eval(get_param(blk, 'bin_pts'));
      | % if (strcmp(mode, 'one value') || strcmp(mode, 'fields of equal size')) && (length(current_bins) > 1),
      | %     error('Only one binary pt may be specified for this mode.');
      | % elseif strcmp(mode, 'fields of arbitrary size')
      | %     current_names = textscan(strtrim(strrep(strrep(get_param(blk, 'names'), ']', ''), '[', '')), '%s');
      | %     current_names = current_names{1};
      | %     numios = length(current_names);
      | %     if length(current_bins) ~= numios,
      | %         error('%d field names specified, but %d binary pts?', numios, length(current_bins));
      | %     end
      | % end
  pof_ddc_I : Subsystem  Tag=xps:sw_reg  AncestorBlock=xps_library/software register  mask(swreg){mode=one value, io_dir=From Processor, io_delay=0, sample_period=1, names=reg, bitwidths=32, arith_types=0, bin_pts=0, sim_port=on, show_format=off}
      mask prompts: io_dir "I/O direction"; io_delay "I/O delay"; sample_period "Sample period"; names "Name:"; bitwidths "Bitwidth:"; arith_types "Type (ufix=0, fix=1, bool=2):"; bin_pts "Binary pt:"; sim_port "Provide sim input/output?"; show_format "Print format string?"
      mask init:
      | swreg_init(gcb)
      settings: AttributesFormatString=1input
      mask TypeOptions mode: one value | fields of equal size | fields of arbitrary size
      mask Callback mode: swreg_cb(gcb);
      mask TypeOptions io_dir: To Processor | From Processor
      mask Callback io_dir:
      | mask_enables = get_param(gcb, 'MaskEnables');
      | mask_names = get_param(gcb, 'MaskNames');
      | if strcmp(get_param(gcb, 'io_dir'), 'To Processor'),
      |     mask_enables{ismember(mask_names, 'sample_period')} = 'off';
      | else
      |     mask_enables{ismember(mask_names, 'sample_period')} = 'on';
      | end
      | set_param(gcb, 'MaskEnables', mask_enables);
      mask Callback bitwidths:
      | swreg_maskcheck(gcb);
      | % blk = gcb;
      | % mode = get_param(blk, 'mode');
      | % current_widths = eval(get_param(blk, 'bitwidths'));
      | % if (strcmp(mode, 'one value') || strcmp(mode, 'fields of equal size')) && (length(current_widths) > 1),
      | %     error('Only one width may be specified for this mode.');
      | % elseif strcmp(mode, 'fields of arbitrary size')
      | %     current_names = textscan(strtrim(strrep(strrep(get_param(blk, 'names'), ']', ''), '[', '')), '%s');
      | %     current_names = current_names{1};
      | %     numios = length(current_names);
      | %     if length(current_widths) ~= numios,
      | %         error('%d field names specified, but %d widths?', numios, length(current_widths));
      | %     end
      | % end
      | % total_width = 0;
      | % for ctr = 1 : length(current_widths),
      | %     total_width = total_width + current_widths(ctr);
      | % end
      | % if total_width > 32,
      | %     error('Total width must be 32 or less, set to %d.', total_width);
      | % end
      mask Callback arith_types:
      | [numios, ~, ~, ~, current_types] = swreg_maskcheck(gcb);
      | % blk = gcb;
      | % mode = get_param(blk, 'mode');
      | % current_types = eval(get_param(blk, 'arith_types'));
      | % numios = length(current_types);
      | % if (strcmp(mode, 'one value') || strcmp(mode, 'fields of equal size')) && (length(current_types) > 1),
      | %     error('Only one type may be specified for this mode.');
      | % elseif strcmp(mode, 'fields of arbitrary size')
      | %     current_names = textscan(strtrim(strrep(strrep(get_param(blk, 'names'), ']', ''), '[', '')), '%s');
      | %     current_names = current_names{1};
      | %     numios = length(current_names);
      | %     if length(current_types) ~= numios,
      | %         error('%d field names specified, but %d types?', numios, length(current_types));
      | %     end
      | % end
      | problem = 0;
      | for ctr = 1 : numios,
      |     t = current_types(ctr);
      |     if (t < 0) || (t > 2),
      |         problem = t;
      |         ctr = numios + 1;
      |     end
      | end
      | if problem ~= 0,
      |     error('Type cannot be %i, must be 0, 1 or 2.', problem);
      | end
      mask Callback bin_pts:
      | swreg_maskcheck(gcb);
      | % blk = gcb;
      | % mode = get_param(blk, 'mode');
      | % current_bins = eval(get_param(blk, 'bin_pts'));
      | % if (strcmp(mode, 'one value') || strcmp(mode, 'fields of equal size')) && (length(current_bins) > 1),
      | %     error('Only one binary pt may be specified for this mode.');
      | % elseif strcmp(mode, 'fields of arbitrary size')
      | %     current_names = textscan(strtrim(strrep(strrep(get_param(blk, 'names'), ']', ''), '[', '')), '%s');
      | %     current_names = current_names{1};
      | %     numios = length(current_names);
      | %     if length(current_bins) ~= numios,
      | %         error('%d field names specified, but %d binary pts?', numios, length(current_bins));
      | %     end
      | % end
  pof_ddc_Q : Subsystem  Tag=xps:sw_reg  AncestorBlock=xps_library/software register  mask(swreg){mode=one value, io_dir=From Processor, io_delay=0, sample_period=1, names=reg, bitwidths=32, arith_types=0, bin_pts=0, sim_port=on, show_format=off}
      mask prompts: io_dir "I/O direction"; io_delay "I/O delay"; sample_period "Sample period"; names "Name:"; bitwidths "Bitwidth:"; arith_types "Type (ufix=0, fix=1, bool=2):"; bin_pts "Binary pt:"; sim_port "Provide sim input/output?"; show_format "Print format string?"
      mask init:
      | swreg_init(gcb)
      settings: AttributesFormatString=1input
      mask TypeOptions mode: one value | fields of equal size | fields of arbitrary size
      mask Callback mode: swreg_cb(gcb);
      mask TypeOptions io_dir: To Processor | From Processor
      mask Callback io_dir:
      | mask_enables = get_param(gcb, 'MaskEnables');
      | mask_names = get_param(gcb, 'MaskNames');
      | if strcmp(get_param(gcb, 'io_dir'), 'To Processor'),
      |     mask_enables{ismember(mask_names, 'sample_period')} = 'off';
      | else
      |     mask_enables{ismember(mask_names, 'sample_period')} = 'on';
      | end
      | set_param(gcb, 'MaskEnables', mask_enables);
      mask Callback bitwidths:
      | swreg_maskcheck(gcb);
      | % blk = gcb;
      | % mode = get_param(blk, 'mode');
      | % current_widths = eval(get_param(blk, 'bitwidths'));
      | % if (strcmp(mode, 'one value') || strcmp(mode, 'fields of equal size')) && (length(current_widths) > 1),
      | %     error('Only one width may be specified for this mode.');
      | % elseif strcmp(mode, 'fields of arbitrary size')
      | %     current_names = textscan(strtrim(strrep(strrep(get_param(blk, 'names'), ']', ''), '[', '')), '%s');
      | %     current_names = current_names{1};
      | %     numios = length(current_names);
      | %     if length(current_widths) ~= numios,
      | %         error('%d field names specified, but %d widths?', numios, length(current_widths));
      | %     end
      | % end
      | % total_width = 0;
      | % for ctr = 1 : length(current_widths),
      | %     total_width = total_width + current_widths(ctr);
      | % end
      | % if total_width > 32,
      | %     error('Total width must be 32 or less, set to %d.', total_width);
      | % end
      mask Callback arith_types:
      | [numios, ~, ~, ~, current_types] = swreg_maskcheck(gcb);
      | % blk = gcb;
      | % mode = get_param(blk, 'mode');
      | % current_types = eval(get_param(blk, 'arith_types'));
      | % numios = length(current_types);
      | % if (strcmp(mode, 'one value') || strcmp(mode, 'fields of equal size')) && (length(current_types) > 1),
      | %     error('Only one type may be specified for this mode.');
      | % elseif strcmp(mode, 'fields of arbitrary size')
      | %     current_names = textscan(strtrim(strrep(strrep(get_param(blk, 'names'), ']', ''), '[', '')), '%s');
      | %     current_names = current_names{1};
      | %     numios = length(current_names);
      | %     if length(current_types) ~= numios,
      | %         error('%d field names specified, but %d types?', numios, length(current_types));
      | %     end
      | % end
      | problem = 0;
      | for ctr = 1 : numios,
      |     t = current_types(ctr);
      |     if (t < 0) || (t > 2),
      |         problem = t;
      |         ctr = numios + 1;
      |     end
      | end
      | if problem ~= 0,
      |     error('Type cannot be %i, must be 0, 1 or 2.', problem);
      | end
      mask Callback bin_pts:
      | swreg_maskcheck(gcb);
      | % blk = gcb;
      | % mode = get_param(blk, 'mode');
      | % current_bins = eval(get_param(blk, 'bin_pts'));
      | % if (strcmp(mode, 'one value') || strcmp(mode, 'fields of equal size')) && (length(current_bins) > 1),
      | %     error('Only one binary pt may be specified for this mode.');
      | % elseif strcmp(mode, 'fields of arbitrary size')
      | %     current_names = textscan(strtrim(strrep(strrep(get_param(blk, 'names'), ']', ''), '[', '')), '%s');
      | %     current_names = current_names{1};
      | %     numios = length(current_names);
      | %     if length(current_bins) ~= numios,
      | %         error('%d field names specified, but %d binary pts?', numios, length(current_bins));
      | %     end
      | % end
  DAC_out : Outport
  chan_data_out : Outport  Port=2
  wires:
  ADC_Q_in/1 -> Register99/1
  Reinterpret29/1 -> Register100/1
  Register101/1 -> Concat7/2
  Register102/1 -> Concat7/1
  Mult0/1 -> Reinterpret31/1
  [reset_dds] -> ddc_q/4
  [reset_dds] -> ddc_I/4
  Constant9/1 -> k/1(sim_1)
  Slice26/1 -> Reinterpret29/1
  k/1(in_reg) -> Slice26/1
  ADC_I_in/1 -> Register98/1
  Register78/1 -> Mult0/1
  ddc_q/2 -> Register92/1
  Constant3/1 -> pof_ddc_I/1(sim_1)
  4tone_FIR4/4 -> Slice25/1
  4tone_FIR4/1 -> Terminator13/1
  Slice24/1 -> Reinterpret28/1
  Slice25/1 -> Reinterpret23/1
  dac_q/2 -> Register90/1
  Mult1/1 -> Reinterpret30/1
  Register91/1 -> mixer/3
  ddc_I/2 -> Register91/1
  Register82/1 -> ddc_q/3
  Register84/1 -> dac_I/2
  dac_I/2 -> Register78/1
  ddc_I/1 -> Terminator10/1
  ddc_q/1 -> Terminator11/1
  Reinterpret24/1 -> Register84/1
  Slice22/1 -> Reinterpret26/1
  Register103/1 -> DAC_out/1
  Register83/1 -> ddc_q/2
  Register87/1 -> dac_q/3
  Register81/1 -> ddc_q/1
  Reinterpret26/1 -> Register88/1
  [reset_dds] -> dac_I/4
  Register92/1 -> mixer/4
  [reset_dds] -> dac_q/4
  Slice21/1 -> Reinterpret25/1
  dac_q/1 -> Terminator9/1
  Register99/1 -> mixer/2
  Register97/1 -> chan_data_out/1
  mixer/2 -> Register94/1
  mixer/1 -> Register95/1
  Concat6/1 -> Register97/1
  Reinterpret23/1 -> Register93/1
  Reinterpret28/1 -> Register96/1
  Register95/1 -> 4tone_FIR4/1
  Register94/1 -> 4tone_FIR4/2
  4tone_FIR4/2 -> Terminator15/1
  Register93/1 -> Concat6/2
  Register96/1 -> Concat6/1
  4tone_FIR4/3 -> Slice24/1
  Register90/1 -> Mult1/1
  Reinterpret31/1 -> Register102/1
  Reinterpret30/1 -> Register101/1
  Register86/1 -> dac_q/2
  Register98/1 -> mixer/1
  Register85/1 -> dac_I/3
  Register89/1 -> ddc_I/3
  Reinterpret27/1 -> Register83/1
  Concat7/1 -> Register103/1
  pof_ddc_I/1(in_reg) -> Slice22/1
  Register88/1 -> ddc_I/2
  Register80/1 -> ddc_I/1
  Register100/1 -> Mult1/2, Mult0/2
  Reinterpret25/1 -> Register86/1
  Reinterpret22/1 -> Register82/1, Register89/1, Register87/1, Register85/1
  Slice23/1 -> Reinterpret27/1
  Constant5/1 -> pof_ddc_Q/1(sim_1)
  pof_ddc_Q/1(in_reg) -> Slice23/1
  Constant1/1 -> pinc/1(sim_1)
  valid_in/1 -> Register81/1, Register80/1, Register79/1, Register77/1
  dac_I/1 -> Terminator14/1
  Slice27/1 -> Reinterpret24/1
  Slice29/1 -> Reinterpret22/1
  Register77/1 -> dac_I/1
  Constant8/1 -> pof_dac_I/1(sim_1)
  pof_dac_I/1(in_reg) -> Slice27/1
  pinc/1(in_reg) -> Slice29/1
  Register79/1 -> dac_q/1
  Constant2/1 -> pof_dac_Q/1(sim_1)
  pof_dac_Q/1(in_reg) -> Slice21/1
